simulink model "milladeregelungauto"  (Simulink 8.6)
settings: Solver=FixedStepDiscrete  StartTime=0.0  StopTime=10.0  RelTol=1e-3
values from neighbouring files (symbols this model uses):
  Battery_SoC_MAX = [0 95]    [milsetupauto.m]
  Battery_Temp_MAX = [0 45]    [milsetupauto.m]
  Battery_Temp_MIN = [0 -5]    [milsetupauto.m]
settings Model: Creator=Natalia.MORENO-MARTI  LastModifiedBy=Natalia.MORENO-MARTI
settings DataIOCC: SaveFormat=Dataset  SignalLoggingSaveFormat=Dataset
settings OptimizationCC: ExpressionDepthLimit=128
settings DebuggingCC: UnderspecifiedInitializationDetection=Simplified  MergeDetectMultiDrivingBlocksExec=error  SolverPrmCheckMsg=none  FcnCallInpInsideContextMsg=EnableAllAsError  StateNameClashWarn=none
settings HardwareCC: ProdBitPerPointer=64  ProdLargestAtomicFloat=Float  ProdIntDivRoundTo=Zero  ProdEndianess=LittleEndian  ProdWordSize=64  ProdHWDeviceType=Intel->x86-64 (Windows64)
settings GRTTargetCC: GeneratePreprocessorConditionals=Use local settings  CombineOutputUpdateFcns=on  GRTInterface=off
settings ConfigComp: CovModelRefEnable=off

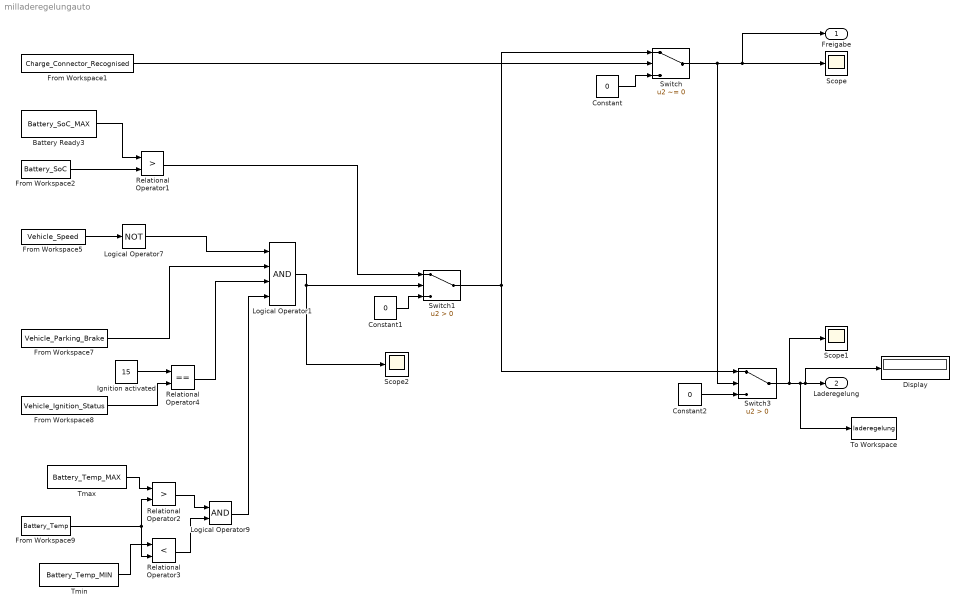
== system milladeregelungauto ==
  Battery Ready3 : Constant  Value=Battery_SoC_MAX
  Constant : Constant  Value=0
  Constant1 : Constant  Value=0
  Constant2 : Constant  Value=0
  Display : Display
  From Workspace1 : FromWorkspace  VariableName=Charge_Connector_Recognised  SampleTime=0
  From Workspace2 : FromWorkspace  VariableName=Battery_SoC  SampleTime=0
  From Workspace5 : FromWorkspace  VariableName=Vehicle_Speed  SampleTime=0
  From Workspace7 : FromWorkspace  VariableName=Vehicle_Parking_Brake  SampleTime=0
  From Workspace8 : FromWorkspace  VariableName=Vehicle_Ignition_Status  SampleTime=0
  From Workspace9 : FromWorkspace  VariableName=Battery_Temp  SampleTime=0
  Ignition activated : Constant  Value=15
  Logical Operator1 : Logic  Inputs=4  AllPortsSameDT=off  OutDataTypeStr=boolean
  Logical Operator7 : Logic  Operator=NOT  AllPortsSameDT=off  OutDataTypeStr=boolean
  Logical Operator9 : Logic  AllPortsSameDT=off  OutDataTypeStr=boolean
  Relational Operator1 : RelationalOperator  Operator=>  OutDataTypeStr=boolean
  Relational Operator2 : RelationalOperator  Operator=>  OutDataTypeStr=boolean
  Relational Operator3 : RelationalOperator  Operator=<  OutDataTypeStr=boolean
  Relational Operator4 : RelationalOperator  Operator===  OutDataTypeStr=boolean
  Scope : Scope
  Scope1 : Scope
  Scope2 : Scope
  Switch : Switch  Criteria=u2 ~= 0
  Switch1 : Switch  Criteria=u2 > Threshold
  Switch3 : Switch  Criteria=u2 > Threshold
  Tmax : Constant  Value=Battery_Temp_MAX
  Tmin : Constant  Value=Battery_Temp_MIN
  To Workspace : ToWorkspace  VariableName=laderegelung  SaveFormat=Timeseries  SampleTime=-1
  Freigabe : Outport
  Laderegelung : Outport  Port=2
  wires:
  From Workspace1/1 -> Switch/2
  Constant/1 -> Switch/3
  Relational Operator1/1 -> Switch1/1
  Switch1/1 -> Switch3/1, Switch/1
  From Workspace5/1 -> Logical Operator7/1
  Logical Operator1/1 -> Scope2/1, Switch1/2
  Constant1/1 -> Switch1/3
  Logical Operator7/1 -> Logical Operator1/1
  From Workspace7/1 -> Logical Operator1/2
  From Workspace9/1 -> Relational Operator3/2, Relational Operator2/2
  Relational Operator2/1 -> Logical Operator9/1
  Relational Operator3/1 -> Logical Operator9/2
  Logical Operator9/1 -> Logical Operator1/4
  Constant2/1 -> Switch3/3
  Switch/1 -> Switch3/2, Freigabe/1, Scope/1
  Switch3/1 -> Scope1/1, To Workspace/1, Display/1, Laderegelung/1
  Tmax/1 -> Relational Operator2/1
  Tmin/1 -> Relational Operator3/1
  From Workspace2/1 -> Relational Operator1/2
  Battery Ready3/1 -> Relational Operator1/1
  Relational Operator4/1 -> Logical Operator1/3
  From Workspace8/1 -> Relational Operator4/2
  Ignition activated/1 -> Relational Operator4/1
